simulink library "tp022479"  (Simulink 6.2)
libraries: simulink3 x3
settings Model: LastModifiedBy=Serg  RTWOptions="-aEnforceIntegerDowncast=1 -aFoldNonRolledExpr=1 -aInlineInvariantSignals=0 -aInlineParameters=0 -aLocalBlockOutputs=1 -aRollThreshold=5 -aGenerateReport=0 -aGenCodeOnly=0 -aRTWVerbose=1 -aIncludeHyperlinkInReport=0 -aLaunchReport=0 -aForceParamTrailComments=0 -aGenerateComments=1 -aIgnoreCustomStorageClasses=1 -aIncHierarchyInIds=0 -aMaxRTWIdLen=31 -aShowEliminatedStatements=0 -aPrefixModelToSubsysFcnNames=1 -aIncDataTypeInIds=0 -aInsertBlockDesc=0 -aSimulinkBlockComments=1 -aInlinedPrmAccess=\"Literals\"  -aSuppressErrorStatus=0 -aModelReferenceCompliant=1 -aSupportNonInlinedSFcns=1 -aSupportContinuousTime=1 -aSupportComplex=1 -aSupportNonFinite=1 -aSupportAbsoluteTime=1 -aTargetPreCompLibLocation=\"\" -aTargetLibSuffix=\"\" -aTargetFcnLib=\"ansi_tfl_tmw.mat\" -aMultiInstanceERTCode=0 -aLogVarNameModifier=\"rt_\" -aIsPILTarget=0 -aCombineOutputUpdateFcns=0 -aGenerateASAP2=0 -aGenerateSampleERTMain=0 -aGenerateFullHeader=1 -aUtilityFuncGeneration=\"Auto\" -aIncludeFileDelimiter=\"Auto\" -aIncludeMdlTerminateFcn=1 -aPurelyIntegerCode=0 -aERTCustomFileBanners=0 -aRTWCAPIStates=0 -aRTWCAPIParams=0 -aRTWCAPISignals=0 -aMatFileLogging=1 -aGenFloatMathFcnCalls=\"ANSI_C\" -aExtModeMexFile=\"ext_comm\" -aExtModeTransport=0 -aExtModeStaticAllocSize=1000000 -aExtModeTesting=0 -aExtModeStaticAlloc=0 -aExtMode=0"

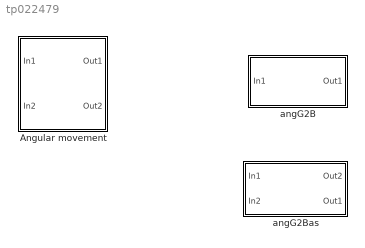
== system tp022479 ==
  Angular movement : Subsystem  SimViewingDevice=off  mask(Angular movement){}
      mask help:
      | Vector VJ=[Jxx, Jyy, Jzz, Jxy, Jyz, Jxz];
      | Ang_g=[fie psi tet];
      mask init:
      | g=(1:40)*pi/30;
      | y=sin(g)/5+0.5;
      | x=cos(g)/5+0.5;
      settings: Permissions=ReadWrite  RTWFcnNameOpts=Auto  RTWFileNameOpts=Auto
      mask Display:
      | port_label('input',1,'M');
      | port_label('input',2,'VJ');
      | port_label('output',1,'Omega');
      | port_label('output',2,'Ang_g');
      | plot(x,y);
      | patch([.64 .75 .69 .64],[.5 .5 .4 .5]);
  angG2B : Subsystem  SimViewingDevice=off
      settings: Permissions=ReadWrite  RTWFcnNameOpts=Auto  RTWFileNameOpts=Auto
      mask Type: angG2B
      mask Description: [fie psi tet]>>>B
      mask Display:
      | port_label('input',1,'Ang_fpt')
      | port_label('output',1,'B')
      | disp('          A_g2B')
  angG2Bas : Subsystem  SimViewingDevice=off
      settings: Permissions=ReadWrite  RTWFcnNameOpts=Auto  RTWFileNameOpts=Auto
      mask Type: angG2Bas
      mask Description: Расчет матрицы B по углам и с-углов
      mask Display:
      | port_label('input',1,'Ang_fpt')
      | port_label('output',2,'B')
      | port_label('output',1,'AngS')
      | disp('Ang2Bas')
      | port_label('input',2,'Bpr')

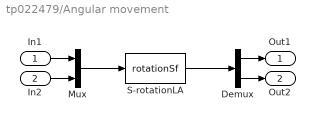
== system tp022479/Angular movement ==
  In1 : Inport  Port=1  PortDimensions=-1  DataType=auto
      settings: SignalType=auto
  In2 : Inport  Port=2  PortDimensions=-1  DataType=auto
      settings: SignalType=auto
  Demux : Demux  Outputs=2  BusSelectionMode=off
  Mux : Mux  Inputs=2  UseBusObject=off
  S-rotationLA : S-Function  FunctionName=rotationSf  Parameters=AnStart  SFunctionModules=''  PortCounts=[]
  Out1 : Outport  Port=1
  Out2 : Outport  Port=2
  wires:
  Mux/1 -> S-rotationLA/1
  S-rotationLA/1 -> Demux/1
  Demux/1 -> Out1/1
  In1/1 -> Mux/1
  Demux/2 -> Out2/1
  In2/1 -> Mux/2

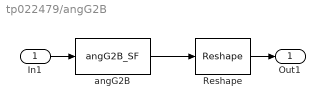
== system tp022479/angG2B ==
  In1 : Inport  Port=1  PortDimensions=-1  DataType=auto
      settings: SignalType=auto
  Reshape : simulink3/Signals & Systems/Reshape  OutputDimensionality=Customize  OutputDimensions=[3,3]
  angG2B : S-Function  FunctionName=angG2B_SF  SFunctionModules=''  PortCounts=[]
  Out1 : Outport  Port=1
  wires:
  angG2B/1 -> Reshape/1
  Reshape/1 -> Out1/1
  In1/1 -> angG2B/1

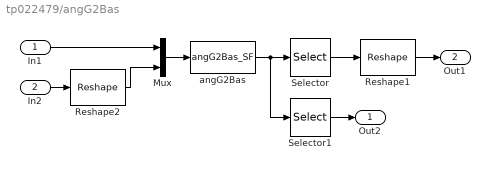
== system tp022479/angG2Bas ==
  In1 : Inport  Port=1  PortDimensions=-1  DataType=auto
      settings: SignalType=auto
  In2 : Inport  Port=2  PortDimensions=-1  DataType=auto
      settings: SignalType=auto
  Mux : Mux  Inputs=2  UseBusObject=off
  Reshape1 : simulink3/Signals & Systems/Reshape  OutputDimensionality=Customize  OutputDimensions=[3,3]
  Reshape2 : simulink3/Signals & Systems/Reshape  OutputDimensionality=Column vector  OutputDimensions=[3,3]
  Selector : Selector  InputType=Vector  ElementSrc=Internal  Elements=[1:9]  RowSrc=Internal  Rows=1  ColumnSrc=Internal  Columns=1  InputPortWidth=12
  Selector1 : Selector  InputType=Vector  ElementSrc=Internal  Elements=[10 :12]  RowSrc=Internal  Rows=1  ColumnSrc=Internal  Columns=1  InputPortWidth=12
  angG2Bas : S-Function  FunctionName=angG2Bas_SF  SFunctionModules=''  PortCounts=[]
  Out2 : Outport  Port=1
  Out1 : Outport  Port=2
  wires:
  angG2Bas/1 -> Selector/1, Selector1/1
  Selector/1 -> Reshape1/1
  Reshape1/1 -> Out1/1
  Selector1/1 -> Out2/1
  In2/1 -> Reshape2/1
  Mux/1 -> angG2Bas/1
  In1/1 -> Mux/1
  Reshape2/1 -> Mux/2
